simulink model "full_code_trim"  (R2014a)
settings: Solver=ode45  StartTime=0.0  StopTime=500.0  RelTol=1e-3
values from neighbouring files (symbols this model uses):
  p_init = 0    [trim_simulate.m]
  phi_init = 0    [trim_simulate.m]
  psi_init = 0    [trim_simulate.m]
  q_init = 0    [trim_simulate.m]
  r_init = 0    [trim_simulate.m]
  theta_init = 0.0105    [trim_simulate.m]
  u_init = 80.00    (= 80)    [trim_simulate.m]
  v_init = 0.00    (= 0)    [trim_simulate.m]
  w_init = 0    [trim_simulate.m]
  xe_init = 0    [trim_simulate.m]
  ye_init = 0    [trim_simulate.m]
  ze_init = -200    [trim_simulate.m]
libraries: aerolibasang x1
settings Model: Creator=sajith  LastModifiedBy=sajith
settings DataIOCC: SignalLoggingSaveFormat=ModelDataLogs
settings OptimizationCC: ExpressionDepthLimit=2147483647
settings DebuggingCC: UnderspecifiedInitializationDetection=Classic  FcnCallInpInsideContextMsg=UseLocalSettings  StateNameClashWarn=warning
settings SFSimCC: SimParseCustomCode=off
settings GRTTargetCC: CombineOutputUpdateFcns=off  GRTInterface=on

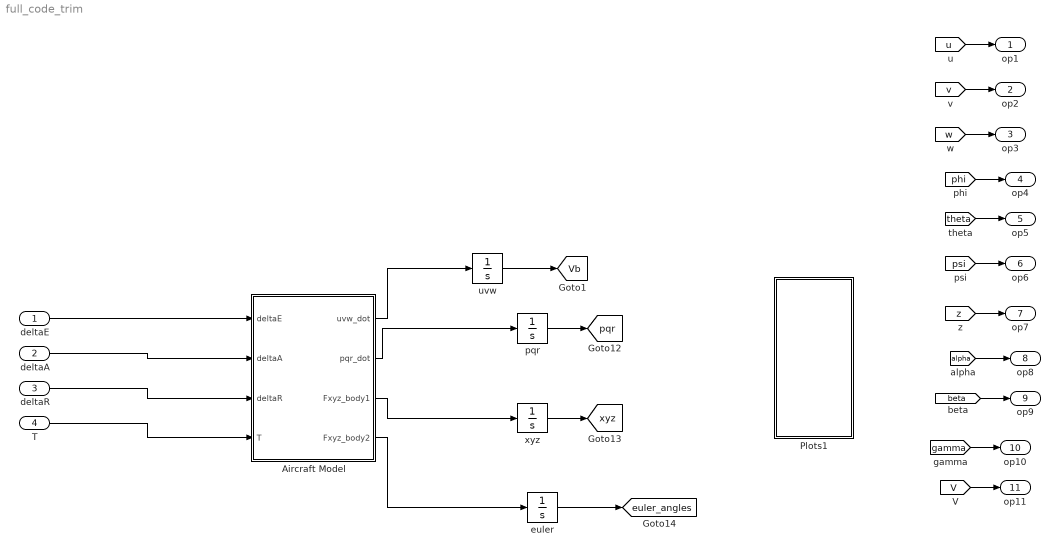
== system full_code_trim ==
  deltaE : Inport
  deltaA : Inport  Port=2
  deltaR : Inport  Port=3
  T : Inport  Port=4
  Aircraft Model : Subsystem
  Plots1 : Subsystem
  euler : Integrator  InitialCondition=[phi_init theta_init psi_init]
  pqr : Integrator  InitialCondition=[p_init q_init r_init]
  uvw : Integrator  InitialCondition=[u_init v_init w_init]
  xyz : Integrator  InitialCondition=[xe_init ye_init ze_init]
  op1 : Outport
  op2 : Outport  Port=2
  op3 : Outport  Port=3
  op4 : Outport  Port=4
  op5 : Outport  Port=5
  op6 : Outport  Port=6
  op7 : Outport  Port=7
  op8 : Outport  Port=8
  op9 : Outport  Port=9
  op10 : Outport  Port=10
  op11 : Outport  Port=11
  tag scope: Vb=global, euler_angles=global, pqr=global, xyz=global
  wires:
  uvw/1 -> [Vb]
  pqr/1 -> [pqr]
  xyz/1 -> [xyz]
  euler/1 -> [euler_angles]
  Aircraft Model/1(uvw_dot) -> uvw/1
  Aircraft Model/2(pqr_dot) -> pqr/1
  Aircraft Model/3(Fxyz_body1) -> xyz/1
  Aircraft Model/4(Fxyz_body2) -> euler/1
  deltaE/1 -> Aircraft Model/1(deltaE)
  T/1 -> Aircraft Model/4(T)
  deltaA/1 -> Aircraft Model/2(deltaA)
  deltaR/1 -> Aircraft Model/3(deltaR)
  [u] -> op1/1
  [v] -> op2/1
  [w] -> op3/1
  [phi] -> op4/1
  [theta] -> op5/1
  [psi] -> op6/1
  [z] -> op7/1
  [alpha] -> op8/1
  [beta] -> op9/1
  [gamma] -> op10/1
  [V] -> op11/1

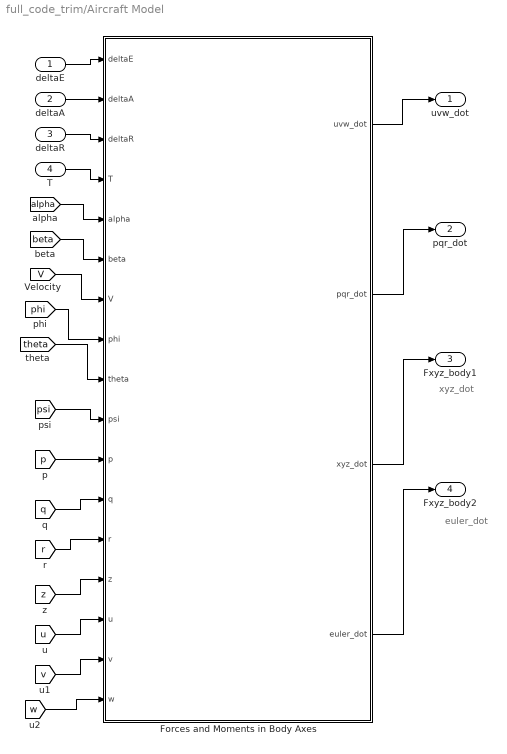
== system full_code_trim/Aircraft Model ==
  note: euler_dot
  note: xyz_dot
  deltaE : Inport
  deltaA : Inport  Port=2
  deltaR : Inport  Port=3
  T : Inport  Port=4
  Forces and Moments in Body Axes : MATLAB Function  TreatAsAtomicUnit=on
  uvw_dot : Outport
  pqr_dot : Outport  Port=2
  Fxyz_body1 : Outport  Port=3
  Fxyz_body2 : Outport  Port=4
  wires:
  [alpha] -> Forces and Moments in Body Axes/5(alpha)
  [beta] -> Forces and Moments in Body Axes/6(beta)
  [V] -> Forces and Moments in Body Axes/7(V)
  [phi] -> Forces and Moments in Body Axes/8(phi)
  [theta] -> Forces and Moments in Body Axes/9(theta)
  [psi] -> Forces and Moments in Body Axes/10(psi)
  [q] -> Forces and Moments in Body Axes/12(q)
  [r] -> Forces and Moments in Body Axes/13(r)
  deltaE/1 -> Forces and Moments in Body Axes/1(deltaE)
  T/1 -> Forces and Moments in Body Axes/4(T)
  deltaA/1 -> Forces and Moments in Body Axes/2(deltaA)
  deltaR/1 -> Forces and Moments in Body Axes/3(deltaR)
  [z] -> Forces and Moments in Body Axes/14(z)
  Forces and Moments in Body Axes/1(uvw_dot) -> uvw_dot/1
  Forces and Moments in Body Axes/2(pqr_dot) -> pqr_dot/1
  Forces and Moments in Body Axes/3(xyz_dot) -> Fxyz_body1/1
  Forces and Moments in Body Axes/4(euler_dot) -> Fxyz_body2/1
  [p] -> Forces and Moments in Body Axes/11(p)
  [u] -> Forces and Moments in Body Axes/15(u)
  [v] -> Forces and Moments in Body Axes/16(v)
  [w] -> Forces and Moments in Body Axes/17(w)

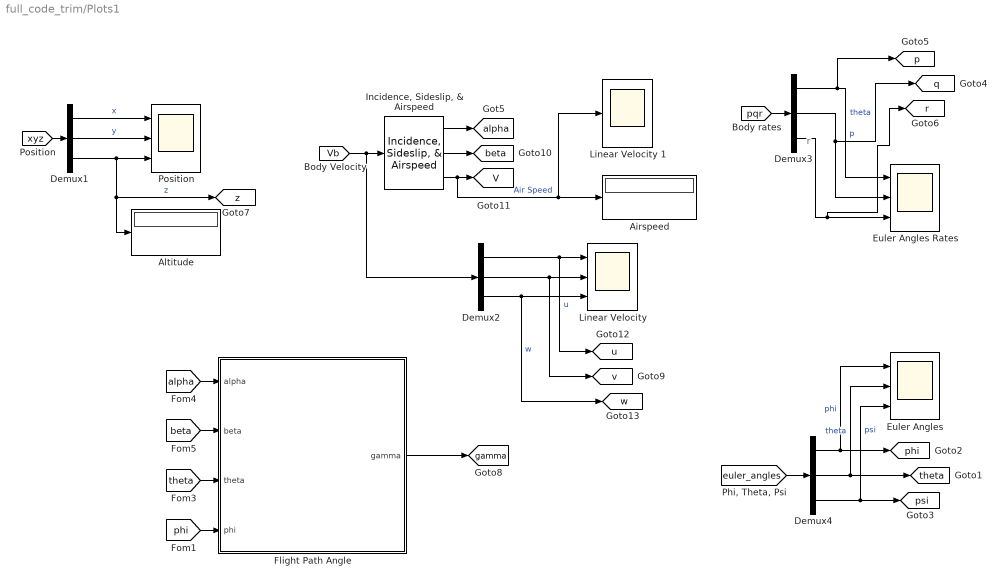
== system full_code_trim/Plots1 ==
  note: r
  Airspeed : Display
  Altitude : Display
  Demux{1..4} (4 alike) : Demux  Outputs=3
  Euler Angles : Scope  NumInputPorts=3
      settings: ShowLegends=on  YMin=-5~-5~-5  YMax=5~5~5  SaveName=ScopeData2
  Euler Angles Rates : Scope  NumInputPorts=3
      settings: ShowLegends=on  YMin=-5~-5~-5  YMax=5~5~5  SaveName=ScopeData3
  Flight Path Angle : MATLAB Function  TreatAsAtomicUnit=on
  "Incidence, Sideslip, & Airspeed" : aerolibasang/Incidence, Sideslip, & Airspeed
  "Linear Velocity " : Scope  NumInputPorts=3
      settings: ShowLegends=on  YMin=-5~-5~-5  YMax=5~5~5  SaveName=ScopeData4
  Linear Velocity 1 : Scope
      settings: ShowLegends=on  SaveName=ScopeData5
  Position : Scope  NumInputPorts=3
      settings: ShowLegends=on  YMin=-5~-5~-5  YMax=5~5~5  SaveName=position
  tag scope: V=global, alpha=global, beta=global, gamma=global, p=global, phi=global, psi=global, q=global, r=global, theta=global, u=global, v=global, w=global, z=global
  wires:
  Demux1/1 -> Position/1  "x"
  Demux1/2 -> Position/2  "y"
  Demux1/3 -> [z], Altitude/1, Position/3  "z"
  Demux2/3 -> [w], "Linear Velocity "/3  "w"
  Demux2/1 -> [u], "Linear Velocity "/1  "u"
  Demux3/1 -> [p], Euler Angles Rates/1  "p"
  Demux4/3 -> [psi], Euler Angles/3  "psi"
  Demux4/2 -> Euler Angles/2, [theta]  "theta"
  Demux4/1 -> Euler Angles/1, [phi]  "phi"
  "Incidence, Sideslip, & Airspeed"/1 -> [alpha]
  "Incidence, Sideslip, & Airspeed"/2 -> [beta]
  "Incidence, Sideslip, & Airspeed"/3 -> [V], Linear Velocity 1/1, Airspeed/1  "Air Speed"
  [xyz] -> Demux1/1
  [euler_angles] -> Demux4/1
  [Vb] -> Demux2/1, "Incidence, Sideslip, & Airspeed"/1
  [pqr] -> Demux3/1
  Demux3/3 -> [r], Euler Angles Rates/3
  Demux3/2 -> [q], Euler Angles Rates/2  "theta"
  [theta] -> Flight Path Angle/3(theta)
  [phi] -> Flight Path Angle/4(phi)
  Flight Path Angle/1(gamma) -> [gamma]
  [alpha] -> Flight Path Angle/1(alpha)
  [beta] -> Flight Path Angle/2(beta)
  Demux2/2 -> [v], "Linear Velocity "/2

== matlab function full_code_trim/Aircraft Model/Forces and Moments in Body Axes ==
  data: deltaE input; uvw_dot output; deltaA input; deltaR input; T input; alpha input; beta input; V input; phi input; theta input; psi input; p input; q input; r input; pqr_dot output; z input; xyz_dot output; euler_dot output; u input; v input; w input
function [uvw_dot,pqr_dot,xyz_dot,euler_dot] = fcn(deltaE,deltaA,deltaR,T,alpha,beta,V,phi,theta,psi,p,q,r,z,u,v,w)
%#codegen

%% environmental constants
g = 9.8; % acceleration due to gravity

%% geometric quantities
c_bar=1.493; % chord length
b=10.911; % wing span
S=16.1651; % wing area

%% mass and inertia
mass = 1043.26; % mass
Ixx=1285.31;
Ixy=0.0;
Iyx=Ixy;
Ixz=0.0;
Izx=Ixz;
Iyy= 1824.93; % moment of inertia
Iyz=0.0;
Izy=Iyz;
Izz=2666.893;

%% aerodynamic coefficients
% drag
cd0=0.036;
cd_alpha = 0.13;
k_drag=0.0830304;
cd_delta_e=0.06;
cd_beta=0.17;

%side force
cy_beta=-0.31;
cy_p=-0.037;
cy_r=0.21;
cy_delta_r=0.187;
cy_delta_a=0;

% lift
cl0=0.25;
cl_alpha=4.47;
cl_q=3.9;
cl_delta_e=0.3476;

% rolling moment
c_l_beta=-0.089;
c_l_p=-0.47;
c_l_r=0.096;
c_l_delta_a=-0.09;
c_l_delta_r=0.0147;

% pitching moment
cm0=-0.02;
cm_alpha=-1.8;
cm_alpha_dot=0.0;
cm_q=-12.4;
cm_delta_e=-1.28;
alpha_dot=0;

% yawing moment
cn_beta=0.065;
cn_p=-0.03;
cn_r=-0.99;
cn_delta_a=-0.0053;
cn_delta_r=-0.0657;



%% Calculations

%%%%%%% Calculation of density with respect to altitude based on ISA
R = 287;
h = -z;  % z direction is downwards

if (h <= 11000)  % temperature gradient region
    Temp = 288.16 - 6.5*10^(-3)*h;
    rho = 1.225 * (Temp/288.16)^(-((g/(-6.5*10^(-3)*R))+1));
    
    
elseif (h > 11000 && h <= 25000) % isothermal region
    rho = 0.3639 * exp(-(g/(R*216.66))*(h-11000));
    

elseif (h > 25000 && h <= 45000) % temperature gradient region
    Temp = 216.66 + 3*10^(-3)*(h-25000);
    rho = 0.03946 * (Temp/216.66)^(-1*((g/(0.003*R))+1));
else 
    rho = 0.08;
end


W = mass*g; %weight

qd = 0.5*rho*V^2; % Dynamic pressure


p_cap = p*b/(2*V);
q_cap = q*c_bar/(2*V);
r_cap = r*b/(2*V);



C_L = cl0+cl_alpha*alpha+cl_q*q_cap+cl_delta_e*deltaE; %coef. of lift
%C_D = cd0+cd_alpha*abs(alpha)+cd_beta*abs(beta)+cd_delta_e*abs(deltaE); % coeff. of drag
C_D = cd0 + k_drag*C_L^2;
C_Y = cy_beta*beta+cy_p*p_cap+cy_r*r_cap+cy_delta_a*deltaA; % coeff. of side slip

% coeff. of moments
C_l = c_l_beta*beta+c_l_p*p_cap+c_l_r*r_cap+c_l_delta_a*deltaA+c_l_delta_r*deltaR; % coeff. of moment about X-axis(tendency to roll)
C_m = cm0 +cm_alpha*alpha+cm_alpha_dot*alpha_dot+cm_delta_e*deltaE; % coeff. of moment about Y-axis(tendency to pitch)
C_n = cn_beta*beta+cn_p*p_cap+cn_r*r_cap+cn_delta_a*deltaA+cn_delta_r*deltaR; % coeff. of moment about Z-axis(tendency to yaw)


%forces
L = qd*S*C_L;
D = qd*S*C_D;
Y = qd*S*C_Y;
W = g*mass;

%moments
l = qd*S*C_l*b;
m = qd*S*C_m*c_bar;
n = qd*S*C_n*b;

%transorm to body axes
trans_wind_body = [cos(alpha)*cos(beta)   -cos(alpha)*sin(beta)   -sin(alpha); ...
    sin(beta)                cos(beta)            0     ; ...
    sin(alpha)*cos(beta)   -sin(alpha)*sin(beta)   cos(alpha)];

forces_body = trans_wind_body*[-D Y -L]' + W*[-sin(theta) sin(phi)*cos(theta) cos(phi)*cos(theta)]' + T*[1 0  0]';

moments_body = [l m n]';


%% Dynamic Equations

% Translation
u_dot = forces_body(1)/mass + r*v - q*w ;
v_dot = forces_body(2)/mass + p*w - r*u ;
w_dot = forces_body(3)/mass + q*u - p*v ;


uvw_dot = [u_dot v_dot w_dot]';

%Rotation
p_dot = (Izz*l + Ixz*n -(Ixz*(Iyy-Ixx-Izz)*p - (Ixz*Ixz+Izz*(Izz-Iyy))*r)*q) / (Ixx*Izz-Ixz*Ixz);
q_dot = m/Iyy - ((Ixx-Izz)/Iyy)*p*r -(Ixz/Iyy)*(p^2 - r^2) ;
r_dot = (Ixz*l + Ixx*n + (Ixz*(Iyy-Ixx-Izz)*r + (Ixz^2+Ixx*(Ixx-Iyy))*p)*q) / (Ixx*Izz-Ixz^2);

pqr_dot = [p_dot q_dot r_dot]';


%% Kinematic Equations 

% Translation - (body to inertial)

xe_dot = u*cos(theta)*cos(psi) + v*(sin(phi)*sin(theta)*cos(psi)-cos(phi)*sin(psi)) + w*(cos(phi)*sin(theta)*cos(psi)+sin(phi)*sin(psi));
ye_dot = u*cos(theta)*sin(psi) + v*(sin(phi)*sin(theta)*sin(psi)+cos(phi)*cos(psi)) + w*(cos(phi)*sin(theta)*sin(psi)-sin(phi)*cos(psi)); 
ze_dot = -u*sin(theta) +  v*sin(phi)*cos(theta) + w*cos(phi)*cos(theta);

xyz_dot = [xe_dot ye_dot ze_dot]';


%Rotation
phi_dot = p+q*sin(phi)*tan(theta) + r*cos(phi)*tan(theta);
theta_dot = q*cos(phi) - r*sin(phi) ;
psi_dot = (q*sin(phi)+r*cos(phi))/cos(theta);

euler_dot = [phi_dot theta_dot psi_dot]';


xdot = [uvw_dot;pqr_dot;xyz_dot;euler_dot];

== matlab function full_code_trim/Plots1/Flight Path Angle ==
  data: alpha input; beta input; theta input; gamma output; phi input
function gamma  = fcn(alpha,beta,theta,phi)
%#codegen

a = cos(alpha)*cos(beta);

b = sin(phi)*sin(beta) + cos(phi)*sin(alpha)*cos(beta);

%theta = (a*b + sin(gamma)*sqrt(a^2 - (sin(gamma))^2 + b^2))/(a^2 - sin(gamma))^2);

gamma = asin(a*sin(theta) - b*cos(theta)); % equation taken from Steven Lewis
